simulink model "linear"  (R2014a)
settings: Solver=ode45  StartTime=0.0  StopTime=0.01  RelTol=1e-3
model workspace (MAT data in the model file):
  Ki = 12447149.4811
  Kd = -86.1936978403
  Kp = 336087.390249
settings Model: CovSFcnEnable=on  Creator=Deadok  LastModifiedBy=User
settings DataIOCC: SignalLoggingSaveFormat=ModelDataLogs
settings OptimizationCC: ExpressionDepthLimit=2147483647  SimCompilerOptimization=off
settings DebuggingCC: AlgebraicLoopMsg=none  UnderspecifiedInitializationDetection=Classic  SolverPrmCheckMsg=none  FcnCallInpInsideContextMsg=UseLocalSettings  UnconnectedInputMsg=none  UnconnectedOutputMsg=none  UnconnectedLineMsg=none  FrameProcessingCompatibilityMsg=error  StateNameClashWarn=warning
settings RTWCC: RTWCompilerOptimization=off
settings GRTTargetCC: CombineOutputUpdateFcns=off  GRTInterface=on

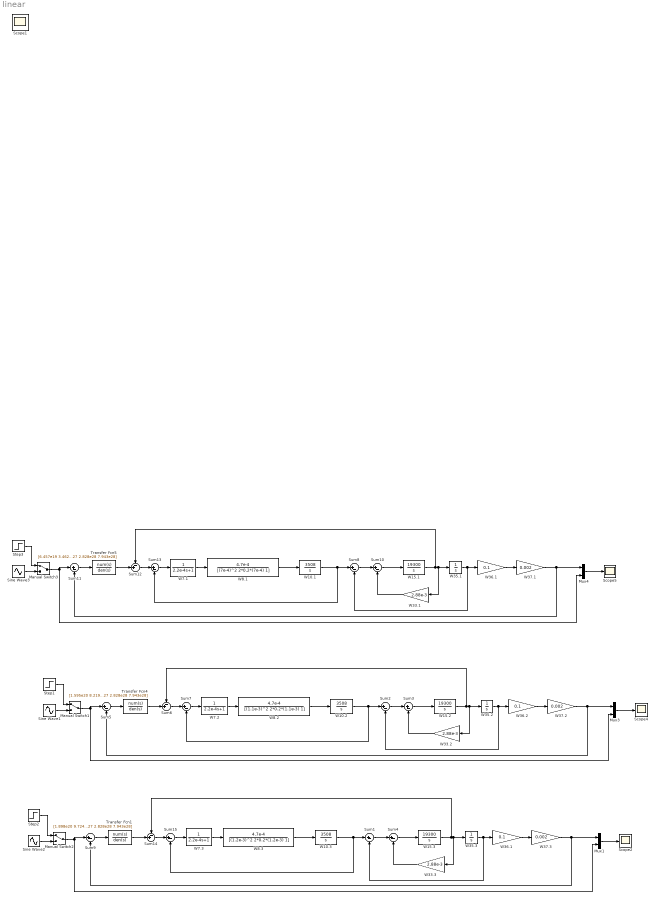
== system linear ==
  Manual Switch1 : ManualSwitch
  Manual Switch2 : ManualSwitch
  Manual Switch3 : ManualSwitch
  Mux1 : Mux  Inputs=2
  Mux3 : Mux  Inputs=2
  Mux4 : Mux  Inputs=2
  Scope{1..2,4..5} (4 alike) : Scope
      Scope2 settings: YMin=1  YMax=1.04
      Scope4 settings: YMin=1  YMax=1.04  SaveName=ScopeData3
      Scope5 settings: YMin=1  YMax=1.04  SaveName=ScopeData4
      Scope1 settings: MaxDataPoints=7500
  Sine Wave1 : Sin  Frequency=3000  SampleTime=0
  Sine Wave2 : Sin  Frequency=3000  SampleTime=0
  Sine Wave3 : Sin  Frequency=3000  SampleTime=0
  Step1 : Step  Time=0  SampleTime=0
  Step2 : Step  Time=0  SampleTime=0
  Step3 : Step  Time=0  SampleTime=0
  Sum{1..5,7..11,13,15} (12 alike) : Sum  Inputs=|+-
  Sum12 : Sum  Inputs=-+|
  Sum14 : Sum  Inputs=-+|
  Sum6 : Sum  Inputs=-+|
  Transfer Fcn1 : TransferFcn  Numerator=[1.898e20 9.724e23 6.525e26 7.317e29 1.642e32 3.673e34 4.914e36 2.854e36]  Denominator=[1 1.539e06 8.565e11 2.152e17 2.439e22 1.001e27 2.828e28 7.943e28]
  Transfer Fcn4 : TransferFcn  Numerator=[1.595e20 8.219e23 5.925e26 7.212e29 1.63e32 3.665e34 4.914e36 2.854e36]  Denominator=[1 1.539e06 8.565e11 2.152e17 2.439e22 1.001e27 2.828e28 7.943e28]
  Transfer Fcn5 : TransferFcn  Numerator=[6.457e19 3.462e23 3.826e26 6.831e29 1.584e32 3.633e34 4.914e36 2.854e36]  Denominator=[1 1.539e06 8.565e11 2.152e17 2.439e22 1.001e27 2.828e28 7.943e28]
  W10.1 : TransferFcn  Numerator=[3508]  Denominator=[1 0]
  W10.2 : TransferFcn  Numerator=[3508]  Denominator=[1 0]
  W10.3 : TransferFcn  Numerator=[3508]  Denominator=[1 0]
  W15.1 : TransferFcn  Numerator=[19300]  Denominator=[1 0]
  W15.2 : TransferFcn  Numerator=[19300]  Denominator=[1 0]
  W15.3 : TransferFcn  Numerator=[19300]  Denominator=[1 0]
  W33.1 : Gain  Gain=2.88e-3  SaturateOnIntegerOverflow=on  OutDataTypeStr=Inherit: Same as input  ParamDataTypeStr=Inherit: Same as input
  W33.2 : Gain  Gain=2.88e-3  SaturateOnIntegerOverflow=on  OutDataTypeStr=Inherit: Same as input  ParamDataTypeStr=Inherit: Same as input
  W33.3 : Gain  Gain=2.88e-3  SaturateOnIntegerOverflow=on  OutDataTypeStr=Inherit: Same as input  ParamDataTypeStr=Inherit: Same as input
  W35.1 : Integrator
  W35.2 : Integrator
  W35.3 : Integrator
  W36.1 : Gain  Gain=0.1
  "W36.1 " : Gain  Gain=0.1
  W36.2 : Gain  Gain=0.1
  W37.1 : Gain  Gain=0.002
  W37.2 : Gain  Gain=0.002
  W37.3 : Gain  Gain=0.002
  W7.1 : TransferFcn  Denominator=[2.2e-4 1]
  W7.2 : TransferFcn  Denominator=[2.2e-4 1]
  W7.3 : TransferFcn  Denominator=[2.2e-4 1]
  W8.1 : TransferFcn  Numerator=[4.7e-4]  Denominator=[(7e-4)^2 2*0.2*(7e-4) 1]
  W8.2 : TransferFcn  Numerator=[4.7e-4]  Denominator=[(1.1e-3)^2 2*0.2*(1.1e-3) 1]
  W8.3 : TransferFcn  Numerator=[4.7e-4]  Denominator=[(1.2e-3)^2 2*0.2*(1.2e-3) 1]
  wires:
  Manual Switch1/1 -> Sum5/1, Mux3/2
  Step1/1 -> Manual Switch1/1
  Sum7/1 -> W7.2/1
  W15.2/1 -> W35.2/1, W33.2/1, Sum6/1
  W7.2/1 -> W8.2/1
  Sine Wave1/1 -> Manual Switch1/2
  Mux3/1 -> Scope4/1
  W33.2/1 -> Sum3/2
  Sum3/1 -> W15.2/1
  Sum2/1 -> Sum3/1
  Sum6/1 -> Sum7/1
  Sum5/1 -> Transfer Fcn4/1
  W10.2/1 -> Sum2/1, Sum7/2
  Transfer Fcn4/1 -> Sum6/2
  W35.2/1 -> W36.2/1, Sum2/2
  W37.2/1 -> Mux3/1, Sum5/2
  W36.2/1 -> W37.2/1
  W8.2/1 -> W10.2/1
  Manual Switch3/1 -> Sum11/1, Mux4/2
  Step3/1 -> Manual Switch3/1
  Sum13/1 -> W7.1/1
  W15.1/1 -> W35.1/1, W33.1/1, Sum12/1
  W7.1/1 -> W8.1/1
  Sine Wave3/1 -> Manual Switch3/2
  Mux4/1 -> Scope5/1
  W33.1/1 -> Sum10/2
  Sum10/1 -> W15.1/1
  Sum8/1 -> Sum10/1
  Sum12/1 -> Sum13/1
  Sum11/1 -> Transfer Fcn5/1
  W10.1/1 -> Sum8/1, Sum13/2
  Transfer Fcn5/1 -> Sum12/2
  W35.1/1 -> "W36.1 "/1, Sum8/2
  W37.1/1 -> Mux4/1, Sum11/2
  "W36.1 "/1 -> W37.1/1
  W8.1/1 -> W10.1/1
  Manual Switch2/1 -> Sum9/1, Mux1/2
  Step2/1 -> Manual Switch2/1
  Sum15/1 -> W7.3/1
  W15.3/1 -> W35.3/1, W33.3/1, Sum14/1
  W7.3/1 -> W8.3/1
  Sine Wave2/1 -> Manual Switch2/2
  Mux1/1 -> Scope2/1
  W33.3/1 -> Sum4/2
  Sum4/1 -> W15.3/1
  Sum1/1 -> Sum4/1
  Sum14/1 -> Sum15/1
  Sum9/1 -> Transfer Fcn1/1
  W10.3/1 -> Sum1/1, Sum15/2
  Transfer Fcn1/1 -> Sum14/2
  W35.3/1 -> W36.1/1, Sum1/2
  W37.3/1 -> Mux1/1, Sum9/2
  W36.1/1 -> W37.3/1
  W8.3/1 -> W10.3/1
